simulink subsystem "lookUpTable"  (R2024a)
settings: Solver=VariableStepAuto  StartTime=0.0  StopTime=10.0  RelTol=1e-3
settings Model: Creator=User  LastModifiedBy=User

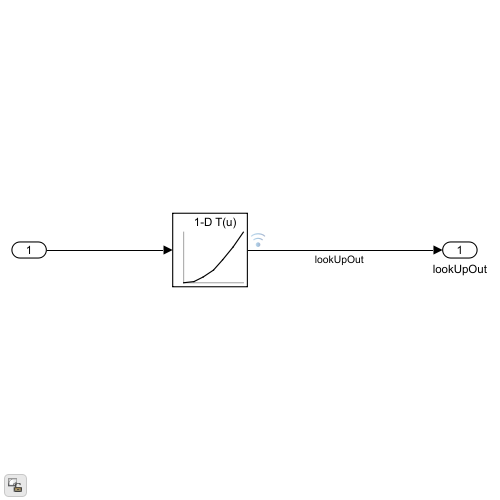
[thumbnail: Simulink's stored preview of the top-level diagram]
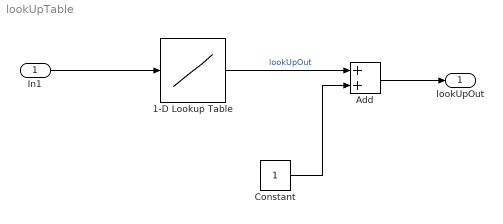
== system lookUpTable ==
  In1 : Inport
  1-D Lookup Table : Lookup_n-D  NumberOfTableDimensions=1  BreakpointsForDimension1=[0 1 2 3 4 5 6]  Table=[0 1 4 9 16 25 36]  InternalRulePriority=Speed  RndMeth=Simplest
  Add : Sum
  Constant : Constant
  lookUpOut : Outport
  wires:
  1-D Lookup Table/1 -> Add/1  "lookUpOut"
  In1/1 -> 1-D Lookup Table/1
  Constant/1 -> Add/2
  Add/1 -> lookUpOut/1
